simulink library "INT_CoVeh_PrfmLim"  (R2016b)
settings: Solver=VariableStepAuto  StartTime=0.0  StopTime=10.0  RelTol=1e-3
settings Model: Creator=Administrator  LastModifiedBy=Administrator

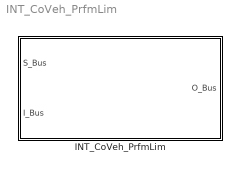
== system INT_CoVeh_PrfmLim ==
  INT_CoVeh_PrfmLim : Subsystem

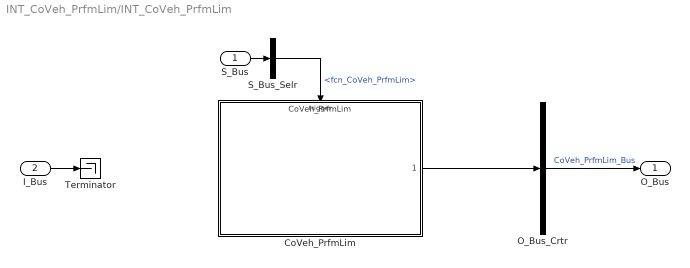
== system INT_CoVeh_PrfmLim/INT_CoVeh_PrfmLim ==
  S_Bus : Inport
  I_Bus : Inport  Port=2
  CoVeh_PrfmLim : ModelReference  ModelNameDialog=CoVeh_PrfmLim  SimulationMode=Normal  ModelReferenceVersion=1.3  TriggerPortName=function  TriggerPortTriggerType=function-call  TriggerPortStatesWhenEnabling=held
  O_Bus_Crtr : BusCreator  Inputs=1
  S_Bus_Selr : BusSelector  OutputSignals=fcn_CoVeh_PrfmLim
  Terminator : Terminator
  O_Bus : Outport
  wires:
  S_Bus_Selr/1 -> CoVeh_PrfmLim/Trigger  "<fcn_CoVeh_PrfmLim>"
  S_Bus/1 -> S_Bus_Selr/1
  I_Bus/1 -> Terminator/1
  O_Bus_Crtr/1 -> O_Bus/1  "CoVeh_PrfmLim_Bus"
  CoVeh_PrfmLim/1 -> O_Bus_Crtr/1
